simulink model "Inverse_matrice22"  (R2022b)
settings: Solver=VariableStepAuto  StartTime=0.0  StopTime=1  RelTol=1e-3
settings Model: Creator=cheye  LastModifiedBy=cheye

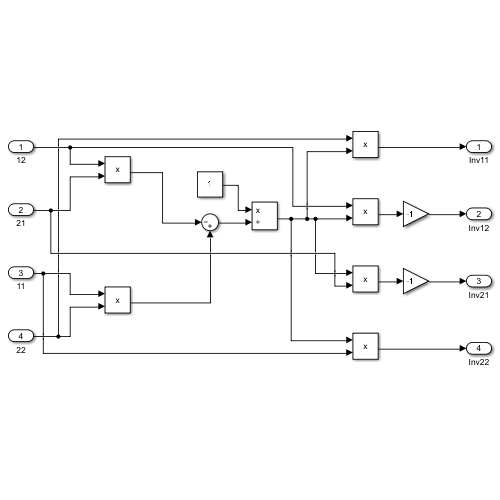
[thumbnail: Simulink's stored preview of the top-level diagram]
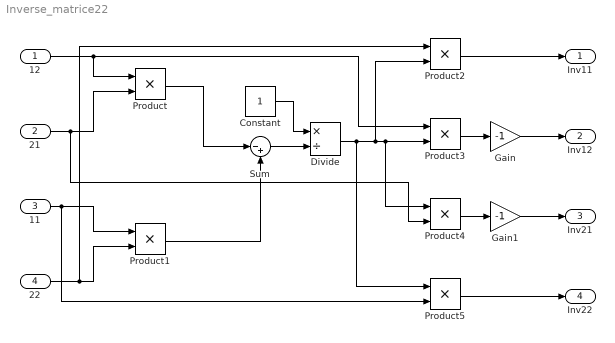
== system Inverse_matrice22 ==
  12 : Inport
  21 : Inport  Port=2
  11 : Inport  Port=3
  22 : Inport  Port=4
  Constant : Constant
  Divide : Product  Inputs=*/
  Gain : Gain  Gain=-1
  Gain1 : Gain  Gain=-1
  Product{,1..5} (6 alike) : Product
  Sum : Sum  Inputs=|-+
  Inv11 : Outport
  Inv12 : Outport  Port=2
  Inv21 : Outport  Port=3
  Inv22 : Outport  Port=4
  wires:
  12/1 -> Product3/1, Product/1
  21/1 -> Product4/2, Product/2
  11/1 -> Product5/2, Product1/1
  22/1 -> Product1/2, Product2/1
  Product/1 -> Sum/1
  Product1/1 -> Sum/2
  Sum/1 -> Divide/2
  Constant/1 -> Divide/1
  Product4/1 -> Gain1/1
  Product3/1 -> Gain/1
  Gain1/1 -> Inv21/1
  Gain/1 -> Inv12/1
  Product5/1 -> Inv22/1
  Product2/1 -> Inv11/1
  Divide/1 -> Product5/1, Product2/2, Product3/2, Product4/1
